simulink model "matlab_node"  (R2025b)
settings: Solver=FixedStepAuto  StartTime=0.0  StopTime=10.0  RelTol=1e-3  SampleTimeConstraint=Specified  EnableMultiTasking=on
undefined symbols (not defined in the file): dt_control, dt_data
libraries: ros2lib x3
settings Model: Creator=vulcangrip  LastModifiedBy=vulcangrip
settings OptimizationCC: DefaultParameterBehavior=Inlined  EnhancedBackFolding=on  PassReuseOutputArgsAs=Individual arguments  ZeroExternalMemoryAtStartup=off  ZeroInternalMemoryAtStartup=off  MaxStackSize=64  OptimizeBlockOrder=speed  DifferentSizesBufferReuse=on  OptimizationCustomize=off  EfficientTunableParamExpr=on
settings DebuggingCC: ParameterTunabilityLossMsg=error
settings HardwareCC: ProdBitPerLong=64.0  ProdLargestAtomicInteger=LongLong  ProdLargestAtomicFloat=Double  ProdLongLongMode=on  ProdHWDeviceType=ARM Compatible->ARM Cortex-A (64-bit)
settings SFSimCC: MATLABDynamicMemAlloc=off  SimTargetLang=C++  SimDLTargetLibrary=mkl-dnn
settings RTWCC: SystemTargetFile=ert.tlc  HardwareBoard=Robot Operating System 2 (ROS 2)  TLCOptions="-aInlineSetEventsForThisBaseRateFcn=TLC_FALSE -aSuppressMultiTaskScheduler=TLC_FALSE  -aRateBasedStepFcn=0"  GenCodeOnly=on  TemplateMakefile=ert_default_tmf  Toolchain=Colcon Tools  TargetLang=C++  Description=Embedded Coder
settings CodeAppCC: ForceParamTrailComments=on  IgnoreCustomStorageClasses=off  OperatorAnnotations=on  SimulinkDataObjDesc=on  SFDataObjDesc=on  InsertBlockDesc=on
settings ERTTargetCC: ExtModeTransport=2.0  ExtModeStaticAlloc=on  ExtModeAutomaticAllocSize=off  ExtModeMexFile=ext_xcp  ExtModeIntrfLevel=Level2 - Open  RootIOFormat=Structure reference  TargetLangStandard=C++11 (ISO)  CodeInterfacePackaging=C++ class  SupportVariableSizeSignals=on

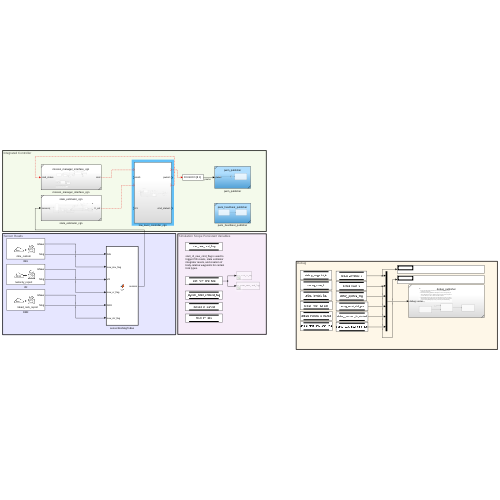
[thumbnail: Simulink's stored preview of the top-level diagram]
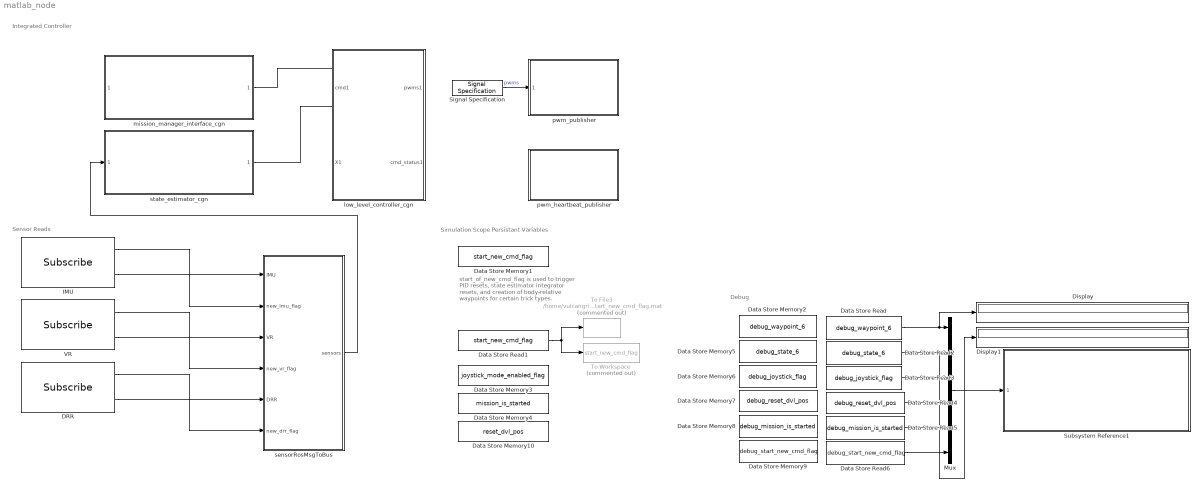
== system matlab_node ==
  note: Integrated Controller
  note: Sensor Reads
  note: Debug
  note: start_of_new_cmd_flag is used to trigger PID resets, state estimator integrator resets, and creation of body-relative waypoints for certain trick types.
  note: Simulation Scope Persistant Variables
  DRR : ros2lib/Subscribe  topicSource=Select from ROS network  topic=/dead_reck_report  messageType=custom_interfaces/DRR  sampleTime=-1  QOSHistory=Keep last  QOSDepth=10  QOSReliability=Reliable  QOSDurability=Volatile  QOSDeadline=Inf  QOSLifespan=Inf  QOSLiveliness=Automatic  QOSLeaseDuration=Inf  QOSAvoidROSNamespaceConventions=off
  Data Store Memory1 : DataStoreMemory  DataStoreName=start_new_cmd_flag  WriteAfterWriteMsg=warning  InitialValue=true  ShowAdditionalParam=off  OutDataTypeStr=boolean
  Data Store Memory10 : DataStoreMemory  DataStoreName=reset_dvl_pos  WriteAfterWriteMsg=warning  InitialValue=false  ShowAdditionalParam=off  OutDataTypeStr=boolean
  Data Store Memory2 : DataStoreMemory  DataStoreName=debug_waypoint_6  WriteAfterWriteMsg=warning  InitialValue=[0 0 0 0 0 0]'  ShowAdditionalParam=off
  Data Store Memory3 : DataStoreMemory  DataStoreName=joystick_mode_enabled_flag  WriteAfterWriteMsg=warning  InitialValue=initial_joystick_mode_enabled_flag  ShowAdditionalParam=off  OutDataTypeStr=boolean
  Data Store Memory4 : DataStoreMemory  DataStoreName=mission_is_started  WriteAfterWriteMsg=warning  InitialValue=false  ShowAdditionalParam=off  OutDataTypeStr=boolean
  Data Store Memory5 : DataStoreMemory  DataStoreName=debug_state_6  WriteAfterWriteMsg=warning  InitialValue=[0 0 0 0 0 0]'  ShowAdditionalParam=off
  Data Store Memory6 : DataStoreMemory  DataStoreName=debug_joystick_flag  WriteAfterWriteMsg=warning  ShowAdditionalParam=off
  Data Store Memory7 : DataStoreMemory  DataStoreName=debug_reset_dvl_pos  WriteAfterWriteMsg=warning  ShowAdditionalParam=off
  Data Store Memory8 : DataStoreMemory  DataStoreName=debug_mission_is_started  WriteAfterWriteMsg=warning  ShowAdditionalParam=off
  Data Store Memory9 : DataStoreMemory  DataStoreName=debug_start_new_cmd_flag  WriteAfterWriteMsg=warning  ShowAdditionalParam=off
  Data Store Read : DataStoreRead  DataStoreName=debug_waypoint_6  IndexOptions=Index vector (dialog)  Indices=1  OutputSizes=1
  Data Store Read1 : DataStoreRead  DataStoreName=start_new_cmd_flag  IndexOptions=Index vector (dialog)  Indices=1  OutputSizes=1
  Data Store Read2 : DataStoreRead  DataStoreName=debug_state_6  IndexOptions=Index vector (dialog)  Indices=1  OutputSizes=1
  Data Store Read3 : DataStoreRead  DataStoreName=debug_joystick_flag  IndexOptions=Index vector (dialog)  Indices=1  OutputSizes=1
  Data Store Read4 : DataStoreRead  DataStoreName=debug_reset_dvl_pos  IndexOptions=Index vector (dialog)  Indices=1  OutputSizes=1
  Data Store Read5 : DataStoreRead  DataStoreName=debug_mission_is_started  IndexOptions=Index vector (dialog)  Indices=1  OutputSizes=1
  Data Store Read6 : DataStoreRead  DataStoreName=debug_start_new_cmd_flag  IndexOptions=Index vector (dialog)  Indices=1  OutputSizes=1
  Display : Display
  Display1 : Display
  IMU : ros2lib/Subscribe  topicSource=Specify your own  topic=/imu_custom  messageType=custom_interfaces/Imu  sampleTime=1/100  QOSHistory=Keep last  QOSDepth=10  QOSReliability=Reliable  QOSDurability=Volatile  QOSDeadline=Inf  QOSLifespan=Inf  QOSLiveliness=Automatic  QOSLeaseDuration=Inf  QOSAvoidROSNamespaceConventions=off
  Mux : Mux  Inputs=6
  Signal Specification : SignalSpecification  OutDataTypeStr=int32  Dimensions=[8 1]
  Subsystem Reference1 : Subsystem  ReferencedSubsystem=debug_publisher
  To File3 : ToFile  Commented=on  Filename=/home/vulcangrip/SimulinkPlant/data/2026_07_06_22_13_57/start_new_cmd_flag.mat  MatrixName=start_new_cmd_flag  SaveFormat=Timeseries
  To Workspace : ToWorkspace  Commented=on  VariableName=start_new_cmd_flag  SaveFormat=Timeseries  SampleTime=dt_data
  VR : ros2lib/Subscribe  topicSource=Select from ROS network  topic=/velocity_report  messageType=custom_interfaces/VR  sampleTime=-1  QOSHistory=Keep last  QOSDepth=10  QOSReliability=Reliable  QOSDurability=Volatile  QOSDeadline=Inf  QOSLifespan=Inf  QOSLiveliness=Automatic  QOSLeaseDuration=Inf  QOSAvoidROSNamespaceConventions=off
  low_level_controller_cgn : Subsystem
  mission_manager_interface_cgn : Subsystem  ReferencedSubsystem=mission_manager_interface_cgn
  pwm_heartbeat_publisher : Subsystem  ReferencedSubsystem=pwm_heartbeat_publisher
  pwm_publisher : Subsystem  ReferencedSubsystem=pwm_publisher
  sensorRosMsgToBus : MATLAB Function  TreatAsAtomicUnit=on
  state_estimator_cgn : Subsystem  ReferencedSubsystem=state_estimator_cgn
  wires:
  VR/2 -> sensorRosMsgToBus/3(VR)
  ? -> Signal Specification/1
  DRR/1 -> sensorRosMsgToBus/6(new_drr_flag)
  VR/1 -> sensorRosMsgToBus/4(new_vr_flag)
  ? -> mission_manager_interface_cgn/1
  state_estimator_cgn/1 -> ?
  IMU/1 -> sensorRosMsgToBus/2(new_imu_flag)
  DRR/2 -> sensorRosMsgToBus/5(DRR)
  sensorRosMsgToBus/1(sensors) -> state_estimator_cgn/1
  mission_manager_interface_cgn/1 -> ?
  Signal Specification/1 -> pwm_publisher/1  "pwms"
  IMU/2 -> sensorRosMsgToBus/1(IMU)
  Data Store Read6/1 -> Mux/6
  Data Store Read5/1 -> Mux/5
  Data Store Read4/1 -> Mux/4
  Mux/1 -> Subsystem Reference1/1
  Data Store Read2/1 -> Display1/1, Mux/2
  Data Store Read/1 -> Display/1, Mux/1
  Data Store Read3/1 -> Mux/3
  Data Store Read1/1 -> To File3/1, To Workspace/1

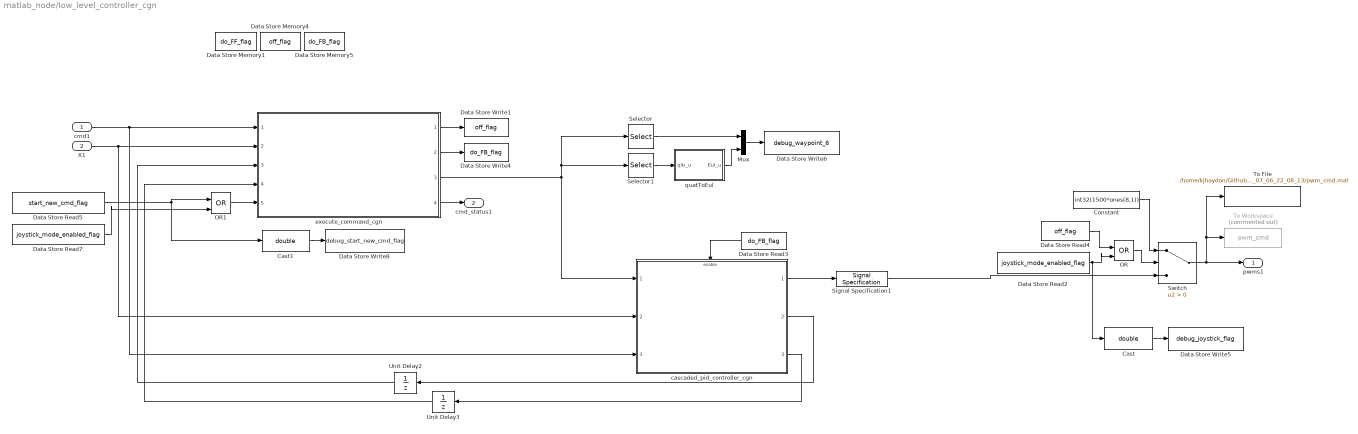
== system matlab_node/low_level_controller_cgn ==
  cmd1 : Inport  OutDataTypeStr=Bus: cmd_bus  SampleTime=dt_control
      settings: VarSizeSig=Yes
  X1 : Inport  Port=2  SampleTime=dt_control
  Cast : DataTypeConversion  OutDataTypeStr=double  SaturateOnIntegerOverflow=off  RndMeth=Floor
  Cast1 : DataTypeConversion  OutDataTypeStr=double  SaturateOnIntegerOverflow=off  RndMeth=Floor
  Constant : Constant  Value=int32(1500*ones(8,1))
  Data Store Memory1 : DataStoreMemory  DataStoreName=do_FF_flag  WriteAfterWriteMsg=warning  ShowAdditionalParam=off
  Data Store Memory4 : DataStoreMemory  DataStoreName=off_flag  WriteAfterWriteMsg=warning  ShowAdditionalParam=off
  Data Store Memory5 : DataStoreMemory  DataStoreName=do_FB_flag  WriteAfterWriteMsg=warning  ShowAdditionalParam=off
  Data Store Read2 : DataStoreRead  DataStoreName=joystick_mode_enabled_flag  IndexOptions=Index vector (dialog)  Indices=1  OutputSizes=1
  Data Store Read3 : DataStoreRead  DataStoreName=do_FB_flag  IndexOptions=Index vector (dialog)  Indices=1  OutputSizes=1
  Data Store Read4 : DataStoreRead  DataStoreName=off_flag  IndexOptions=Index vector (dialog)  Indices=1  OutputSizes=1
  Data Store Read5 : DataStoreRead  DataStoreName=start_new_cmd_flag  IndexOptions=Index vector (dialog)  Indices=1  OutputSizes=1
  Data Store Read7 : DataStoreRead  DataStoreName=joystick_mode_enabled_flag  IndexOptions=Index vector (dialog)  Indices=1  OutputSizes=1
  Data Store Write1 : DataStoreWrite  DataStoreName=off_flag  IndexOptions=Index vector (dialog)  Indices=1  OutputSizes=1
  Data Store Write4 : DataStoreWrite  DataStoreName=do_FB_flag  IndexOptions=Index vector (dialog)  Indices=1  OutputSizes=1
  Data Store Write5 : DataStoreWrite  DataStoreName=debug_joystick_flag  IndexOptions=Index vector (dialog)  Indices=1  OutputSizes=1
  Data Store Write6 : DataStoreWrite  DataStoreName=debug_waypoint_6  IndexOptions=Index vector (dialog)  Indices=1  OutputSizes=1
  Data Store Write8 : DataStoreWrite  DataStoreName=debug_start_new_cmd_flag  IndexOptions=Index vector (dialog)  Indices=1  OutputSizes=1
  Mux : Mux  Inputs=2
  OR : Logic  Operator=OR  IconShape=distinctive  AllPortsSameDT=off  OutDataTypeStr=boolean
  OR1 : Logic  Operator=OR  IconShape=distinctive  AllPortsSameDT=off  OutDataTypeStr=boolean
  Selector : Selector  InputPortWidth=13  IndexOptions=Index vector (dialog)  Indices=[1 2 3]  OutputSizes=1
  Selector1 : Selector  InputPortWidth=13  IndexOptions=Index vector (dialog)  Indices=[4 5 6 7]  OutputSizes=1
  Signal Specification1 : SignalSpecification  OutDataTypeStr=int32
  Switch : Switch  Criteria=u2 > Threshold  SaturateOnIntegerOverflow=off  InputSameDT=off
  To File : ToFile  Filename=/home/kjhaydon/Github/Robosub/SimulinkPlant/data/2026_07_06_22_08_13/pwm_cmd.mat  MatrixName=pwm_cmd  SaveFormat=Timeseries  SampleTime=dt_data
  To Workspace : ToWorkspace  Commented=on  VariableName=pwm_cmd  SaveFormat=Timeseries  SampleTime=dt_data
  Unit Delay2 : UnitDelay  SampleTime=dt_control  HasFrameUpgradeWarning=on
  Unit Delay3 : UnitDelay  SampleTime=dt_control  HasFrameUpgradeWarning=on
  cascaded_pid_controller_cgn : Subsystem  ReferencedSubsystem=cascaded_pid_controller_cgn
  execute_command_cgn : Subsystem  ReferencedSubsystem=execute_command_cgn
  quatToEul : MATLAB Function  TreatAsAtomicUnit=on
  pwms1 : Outport
  cmd_status1 : Outport  Port=2  SampleTime=dt_control
  wires:
  cmd1/1 -> cascaded_pid_controller_cgn/3, execute_command_cgn/1
  Mux/1 -> Data Store Write6/1
  cascaded_pid_controller_cgn/3 -> Unit Delay3/1
  Constant/1 -> Switch/1
  execute_command_cgn/1 -> Data Store Write1/1
  Unit Delay2/1 -> execute_command_cgn/3
  Cast1/1 -> Data Store Write8/1
  X1/1 -> cascaded_pid_controller_cgn/2, execute_command_cgn/2
  OR1/1 -> execute_command_cgn/5
  execute_command_cgn/3 -> cascaded_pid_controller_cgn/1, Selector/1, Selector1/1
  Data Store Read2/1 -> Cast/1, OR/2
  Cast/1 -> Data Store Write5/1
  Switch/1 -> To Workspace/1, To File/1, pwms1/1
  Data Store Read3/1 -> cascaded_pid_controller_cgn/Enable
  quatToEul/1(Eul_u) -> Mux/2
  execute_command_cgn/2 -> Data Store Write4/1
  Signal Specification1/1 -> Switch/3
  cascaded_pid_controller_cgn/2 -> Unit Delay2/1
  execute_command_cgn/4 -> cmd_status1/1
  Data Store Read5/1 -> OR1/1, Cast1/1
  Data Store Read7/1 -> OR1/2
  Data Store Read4/1 -> OR/1
  OR/1 -> Switch/2
  Selector1/1 -> quatToEul/1(qib_u)
  Unit Delay3/1 -> execute_command_cgn/4
  cascaded_pid_controller_cgn/1 -> Signal Specification1/1
  Selector/1 -> Mux/1

== matlab function matlab_node/sensorRosMsgToBus ==
  data: IMU input Bus: SL_Bus_custom_interfaces_Imu; new_imu_flag input; sensors output Bus: sensor_bus; VR input Bus: SL_Bus_custom_interfaces_VR; new_vr_flag input; DRR input Bus: SL_Bus_custom_interfaces_DRR size=[1,1]; new_drr_flag input
function sensors = fcn(IMU, new_imu_flag, VR, new_vr_flag, DRR, new_drr_flag)

sensors = sensorRosMsgToBus(IMU, new_imu_flag, VR, new_vr_flag, DRR, new_drr_flag);

== matlab function matlab_node/low_level_controller_cgn/quatToEul ==
  data: qib_u input; Eul_u output
function Eul_u = fcn(qib_u)

Eul_u = quatToEul(qib_u);
